simulink model "LiquidLevelSystemWithoutPID"  (R2020b)
settings: Solver=ode45  StartTime=0.0  StopTime=500  RelTol=1e-3  EnableMultiTasking=on
PreLoadFcn:
  | Initialize
StopFcn:
  | Plot_and_save
undefined symbols (not defined in the file or in its folder): P, PlotTanks
libraries: simulink x3
settings Model: Creator=tsladeche  LastModifiedBy=dalal
settings DataIOCC: LimitDataPoints=on  SaveFormat=Array  SignalLoggingSaveFormat=ModelDataLogs  ReturnWorkspaceOutputs=off
settings OptimizationCC: ExpressionDepthLimit=2147483647  LifeSpan=inf
settings DebuggingCC: UnderspecifiedInitializationDetection=Classic  MergeDetectMultiDrivingBlocksExec=none  SolverPrmCheckMsg=warning  FcnCallInpInsideContextMsg=warning  StateNameClashWarn=warning  SFUnexpectedBacktrackingDiag=warning  SFNoUnconditionalDefaultTransitionDiag=warning  SFExecutionAtInitializationDiag=none  ArithmeticOperatorsInVariantConditions=warning
settings HardwareCC: ProdBitPerPointer=32  ProdBitPerSizeT=32  ProdBitPerPtrDiffT=32  ProdLargestAtomicFloat=None  ProdIntDivRoundTo=Undefined  ProdEndianess=Unspecified  ProdWordSize=32  ProdHWDeviceType=32-bit Generic
settings ModelReferenceCC: PropagateSignalLabelsOutOfModel=off
settings SFSimCC: SimUseLocalCustomCode=off  CustomCodeUndefinedFunction=UseInterfaceOnly
settings RTWCC: RTWUseLocalCustomCode=off
settings CodeAppCC: StateflowObjectComments=on
settings GRTTargetCC: TargetLangStandard=C89/C90 (ANSI)  CombineOutputUpdateFcns=off  GRTInterface=on
settings ConfigComp: CovMetricSettings=dw  CovSaveCumulativeToWorkspaceVar=on  CovSaveSingleToWorkspaceVar=on  CovExternalEMLEnable=off  CovSFcnEnable=off

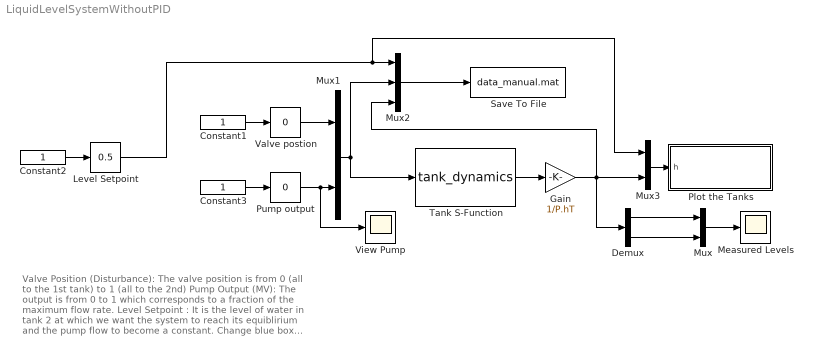
== system LiquidLevelSystemWithoutPID ==
  note: Valve Position (Disturbance): The valve position is from
      | 0 (all to the 1st tank) to 1 (all to the 2nd)
      |
      | Pump Output (MV): The output is from 0 to 1 which
      | corresponds to a fraction of the maximum flow rate.
      |
      | Level Setpoint : It is the level of water in tank 2 at which
      | we want the system to reach its equiblirium and the pump
      | flow to become a constant.
      |
      | Change blue box values (slider).
  Constant1 : Constant
  Constant2 : Constant
  Constant3 : Constant
  Demux : Demux  Outputs=2
  Gain : Gain  Gain=1/P.hT
  Level Setpoint : simulink/Math Operations/Slider Gain  gain=0.5  low=0  high=1
  Measured Levels : Scope
  Mux : Mux  Inputs=2
  Mux1 : Mux  Inputs=2
  Mux2 : Mux  Inputs=3
  Mux3 : Mux  Inputs=2
  Plot the Tanks : Subsystem
  Pump output : simulink/Math Operations/Slider Gain  gain=0  low=0  high=1
  Save To File : ToFile  Filename=data_manual.mat  MatrixName=tanks  SampleTime=1
  Tank S-Function : S-Function  FunctionName=tank_dynamics  Parameters=P  SFunctionDeploymentMode=off  EnableBusSupport=off
  Valve postion : simulink/Math Operations/Slider Gain  gain=0  low=0  high=1
  View Pump : Scope
  wires:
  Gain/1 -> Mux3/2, Demux/1, Mux2/3
  Tank S-Function/1 -> Gain/1
  Constant3/1 -> Pump output/1
  Mux2/1 -> Save To File/1
  Constant1/1 -> Valve postion/1
  Mux1/1 -> Mux2/2, Tank S-Function/1
  Pump output/1 -> View Pump/1, Mux1/2
  Valve postion/1 -> Mux1/1
  Constant2/1 -> Level Setpoint/1
  Level Setpoint/1 -> Mux3/1, Mux2/1
  Mux3/1 -> Plot the Tanks/1(h)
  Mux/1 -> Measured Levels/1
  Demux/1 -> Mux/1
  Demux/2 -> Mux/2

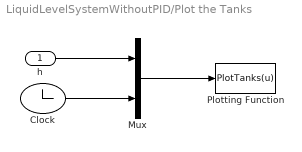
== system LiquidLevelSystemWithoutPID/Plot the Tanks ==
  h : Inport
  Clock : Clock
  Mux : Mux  Inputs=2
  Plotting Function : MATLABFcn  MATLABFcn=PlotTanks(u)  OutputDimensions=0  SampleTime=.05
  wires:
  Mux/1 -> Plotting Function/1
  Clock/1 -> Mux/2
  h/1 -> Mux/1
